simulink model "dynamics_standard_block_CHECK"  (R2017b)
settings: Solver=ode45  StartTime=0.0  StopTime=10  RelTol=1e-3  EnableMultiTasking=on
settings Model: Creator=sagl_ma  LastModifiedBy=hazr_sh
settings DataIOCC: LimitDataPoints=on  SaveFormat=Array
settings OptimizationCC: LifeSpan=inf
settings DebuggingCC: SFUnexpectedBacktrackingDiag=warning  SFNoUnconditionalDefaultTransitionDiag=warning  SFExecutionAtInitializationDiag=none
settings HardwareCC: ProdBitPerPointer=32  ProdBitPerSizeT=32  ProdBitPerPtrDiffT=32  ProdLargestAtomicFloat=None  ProdIntDivRoundTo=Undefined  ProdEndianess=Unspecified  ProdWordSize=32  ProdHWDeviceType=32-bit Generic
settings ModelReferenceCC: PropagateSignalLabelsOutOfModel=off
settings CodeAppCC: StateflowObjectComments=on
settings GRTTargetCC: TargetLangStandard=C89/C90 (ANSI)  GeneratePreprocessorConditionals=Disable all
settings ConfigComp: CovMetricSettings=dw  CovHtmlReporting=on  CovSaveCumulativeToWorkspaceVar=on  CovSaveSingleToWorkspaceVar=on  CovExternalEMLEnable=off

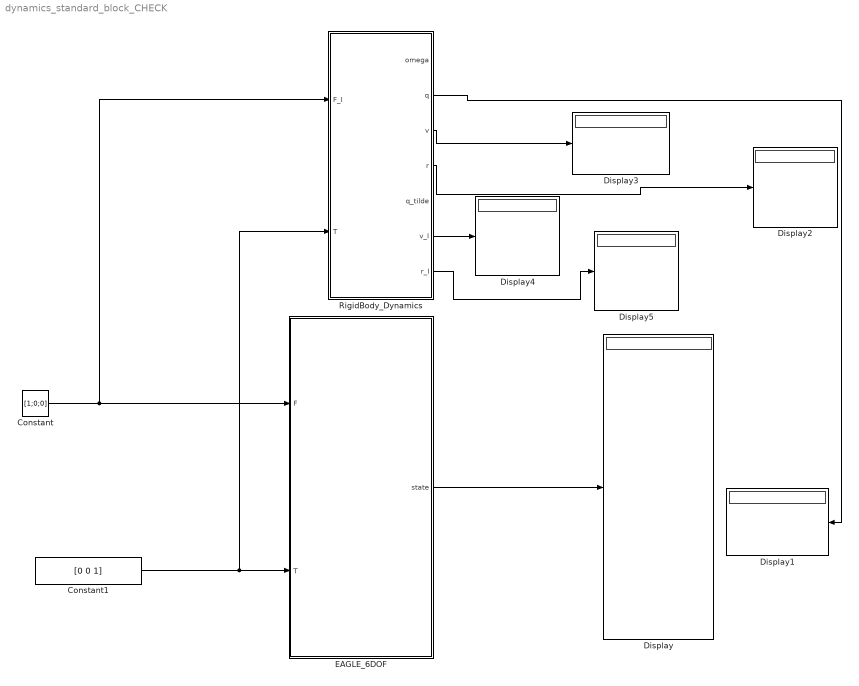
== system dynamics_standard_block_CHECK ==
  Constant : Constant  Value=[1;0;0]
  Constant1 : Constant  Value=[0 0 1]
  Display{,1..5} (6 alike) : Display
  EAGLE_6DOF : Subsystem  mask{r0=[0;0;0], v0=[0;0;0], m0=1, q_I_B0=[0;0;0;1], omega0=[0;0;0], I0=eye(3)}
      mask prompts: r0 "Initial position (m) in inertial reference frame, [3,1]"; v0 "Initial velocity (m/s) in inertial reference frame, [3,1]"; m0 "Initial mass (kg), [1,1]"; q_I_B0 "Initial quaternion defining the orientation from inertial reference frame to body reference frame [4,1]"; omega0 "Initial angular velocity (rad/s) in body reference frame, [3,1]"; I0 "Initial Inertia matrix (kg*m2),  [3,3]"
  RigidBody_Dynamics : Subsystem  mask{r0=[0;0;0], v0=[0;0;0], m0=1, q0=[0;0;0;1], w0=[0;0;0], J0=eye(3)}
      mask prompts: r0 "Initial position (m) in inertial reference frame, [3,1]"; v0 "Initial velocity (m/s) in inertial reference frame, [3,1]"; m0 "Initial mass (kg), [1,1]"; q0 "Initial quaternion defining the orientation in body reference frame [4,1]"; w0 "Initial angular velocity (rad/s) in body reference frame, [3,1]"; J0 "Initial Inertia matrix (kg*m2),  [3,3]"
  wires:
  Constant/1 -> RigidBody_Dynamics/1(F_I), EAGLE_6DOF/1(F)
  Constant1/1 -> RigidBody_Dynamics/2(T), EAGLE_6DOF/2(T)
  EAGLE_6DOF/1(state) -> Display/1
  RigidBody_Dynamics/2(q) -> Display1/1
  RigidBody_Dynamics/4(r) -> Display2/1
  RigidBody_Dynamics/3(v) -> Display3/1
  RigidBody_Dynamics/6("v_I ") -> Display4/1
  RigidBody_Dynamics/7(r_I) -> Display5/1

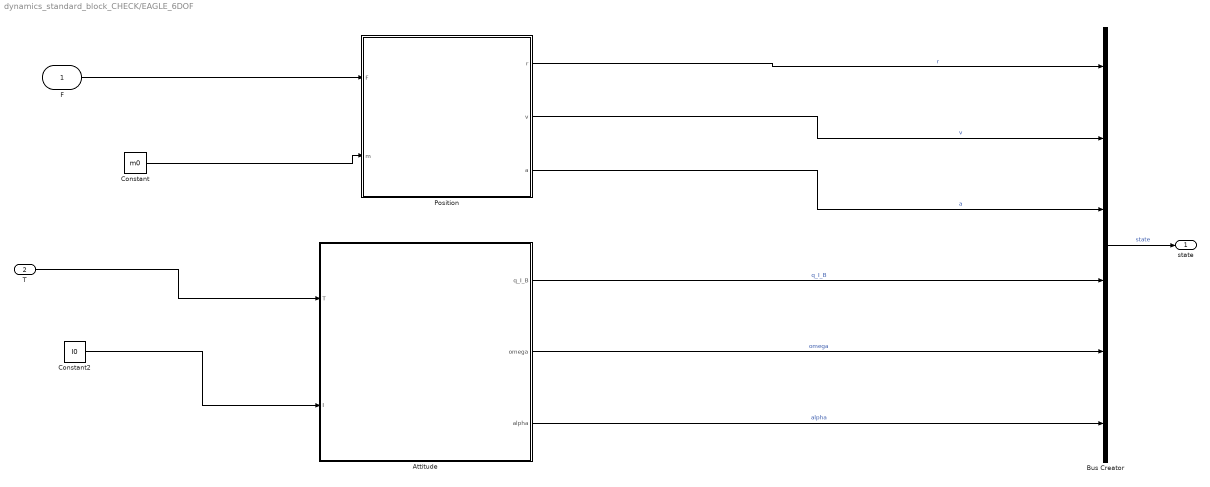
== system dynamics_standard_block_CHECK/EAGLE_6DOF ==
  F : Inport
  T : Inport  Port=2
  Attitude : Subsystem
  Bus Creator : BusCreator  Inputs=6
  Constant : Constant  Value=m0
  Constant2 : Constant  Value=I0
  Position : Subsystem
  state : Outport
  wires:
  Constant2/1 -> Attitude/2(I)
  Attitude/3(alpha) -> Bus Creator/6  "alpha"
  Attitude/2(omega) -> Bus Creator/5  "omega"
  Attitude/1(q_I_B) -> Bus Creator/4  "q_I_B"
  Position/3(a) -> Bus Creator/3  "a"
  Position/1(r) -> Bus Creator/1  "r"
  Position/2(v) -> Bus Creator/2  "v"
  Bus Creator/1 -> state/1  "state"
  Constant/1 -> Position/2(m)
  F/1 -> Position/1(F)
  T/1 -> Attitude/1(T)

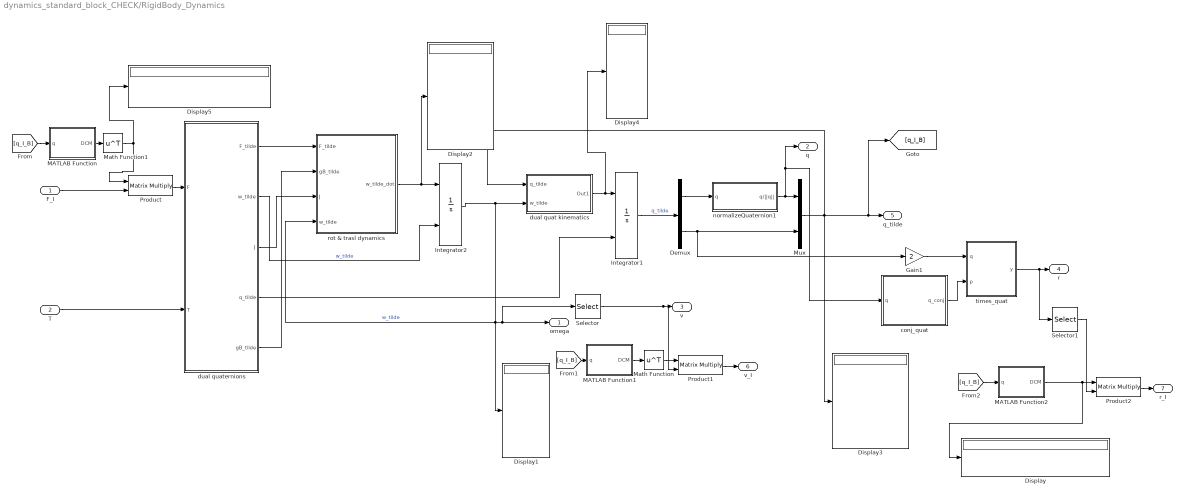
== system dynamics_standard_block_CHECK/RigidBody_Dynamics ==
  F_I : Inport
  T : Inport  Port=2
  Demux : Demux  Outputs=2
  Display{,1..5} (6 alike) : Display
  Gain1 : Gain  Gain=2
  Integrator1 : Integrator  InitialConditionSource=external
  Integrator2 : Integrator  InitialConditionSource=external
  MATLAB Function : MATLAB Function  TreatAsAtomicUnit=on
  MATLAB Function1 : MATLAB Function  TreatAsAtomicUnit=on
  MATLAB Function2 : MATLAB Function  TreatAsAtomicUnit=on
  Math Function : Math  Operator=transpose  SaturateOnIntegerOverflow=on
  Math Function1 : Math  Operator=transpose  SaturateOnIntegerOverflow=on
  Mux : Mux  Inputs=[4,4]
  Product : Product  Multiplication=Matrix(*)
  Product1 : Product  Multiplication=Matrix(*)
  Product2 : Product  Multiplication=Matrix(*)
  Selector : Selector  InputPortWidth=8  IndexOptions=Index vector (dialog)  Indices=[5:7]  OutputSizes=1
  Selector1 : Selector  InputPortWidth=4  IndexOptions=Index vector (dialog)  Indices=[1:3]  OutputSizes=1
  conj_quat : MATLAB Function  TreatAsAtomicUnit=on
  dual quat kinematics : Subsystem
  dual quaternions : Subsystem
  normalizeQuaternion1 : Subsystem  mask(normalizeQuaternion){}
      mask help:
      | This block is normalizing a quaternion. It changes a any quaternion into a
      | unit quaternion.
      |
      | Input:
      | 1) four dimensional quaternion
      |
      | Output:
      | 1) four dimensional unit quaternion
      mask Help: web(which('HPS_mathematics_lib-normalizeQuaternion.html'),'-helpbrowser')
  rot & trasl dynamics : Subsystem
  times_quat : MATLAB Function  TreatAsAtomicUnit=on
  omega : Outport
  q : Outport  Port=2
  v : Outport  Port=3
  r : Outport  Port=4
  "q_tilde " : Outport  Port=5
  "v_I " : Outport  Port=6
  r_I : Outport  Port=7
  wires:
  dual quaternions/1(F_tilde) -> rot & trasl dynamics/1(F_tilde)
  dual quaternions/5(gB_tilde) -> rot & trasl dynamics/2(gB_tilde)
  dual quaternions/3(J) -> rot & trasl dynamics/3(J)
  rot & trasl dynamics/1(w_tilde_dot) -> Display2/1, Integrator2/1
  Integrator2/1 -> Display1/1, Selector/1, omega/1, rot & trasl dynamics/4(w_tilde), dual quat kinematics/2(w_tilde)  "w_tilde"
  dual quat kinematics/1(Out1) -> Display4/1, Integrator1/1
  dual quaternions/2(w_tilde) -> Integrator2/2  "w_tilde"
  dual quaternions/4(q_tilde) -> Integrator1/2
  Demux/1 -> normalizeQuaternion1/1(q)
  Integrator1/1 -> Demux/1  "q_tilde"
  Demux/2 -> Gain1/1, Mux/2
  Gain1/1 -> times_quat/1(q)
  Mux/1 -> dual quat kinematics/1(q_tilde), Display3/1, "q_tilde "/1, [q_I_B]
  [q_I_B] -> MATLAB Function/1(q)
  F_I/1 -> Product/2
  Product/1 -> dual quaternions/1(F)
  normalizeQuaternion1/1(q/||q||) -> conj_quat/1(q), q/1, Mux/1
  conj_quat/1(q_conj) -> times_quat/2(p)
  times_quat/1(y) -> Selector1/1, r/1
  [q_I_B] -> MATLAB Function1/1(q)
  MATLAB Function1/1(DCM) -> Math Function/1
  Selector/1 -> Product1/2, v/1
  Math Function/1 -> Product1/1
  Product1/1 -> "v_I "/1
  [q_I_B] -> MATLAB Function2/1(q)
  Product2/1 -> r_I/1
  Selector1/1 -> Product2/2
  MATLAB Function2/1(DCM) -> Display/1, Product2/1
  MATLAB Function/1(DCM) -> Math Function1/1
  Math Function1/1 -> Product/1, Display5/1
  T/1 -> dual quaternions/2(T)

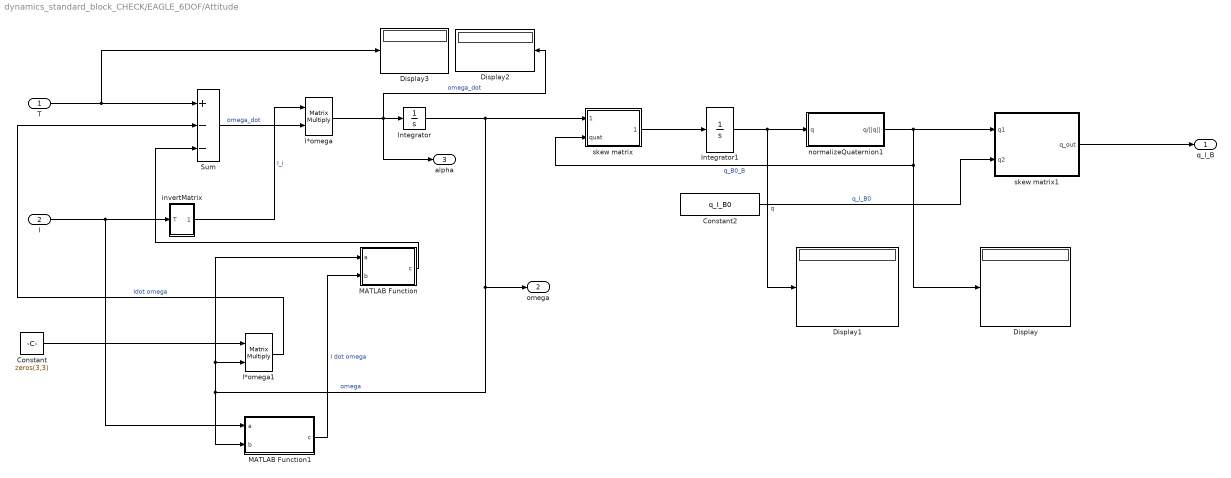
== system dynamics_standard_block_CHECK/EAGLE_6DOF/Attitude ==
  T : Inport
  I : Inport  Port=2
  Constant : Constant  Value=zeros(3,3)
  Constant2 : Constant  Value=q_I_B0
  Display{,1..3} (4 alike) : Display
  I*omega : Product  Multiplication=Matrix(*)  RndMeth=Zero
  I*omega1 : Product  Multiplication=Matrix(*)  RndMeth=Zero
  Integrator : Integrator  InitialCondition=omega0
  Integrator1 : Integrator  InitialCondition=[0;0;0;1]
  MATLAB Function : MATLAB Function  TreatAsAtomicUnit=on
  MATLAB Function1 : MATLAB Function  TreatAsAtomicUnit=on
  Sum : Sum  Inputs=+--
  invertMatrix : Subsystem  mask(invertMatrix){}
      mask help:
      | This block inverts a matrix.
      |
      | Input:
      |     T: [3 x 3] matrix
      |
      | Output:
      |     T_inv: [3 x 3] inverted matrix
      mask Help: web(which('HPS_mathematics_lib-invertMatrix.html'),'-helpbrowser')
  normalizeQuaternion1 : Subsystem  mask(normalizeQuaternion){}
      mask help:
      | This block is normalizing a quaternion. It changes a any quaternion into a
      | unit quaternion.
      |
      | Input:
      | 1) four dimensional quaternion
      |
      | Output:
      | 1) four dimensional unit quaternion
      mask Help: web(which('HPS_mathematics_lib-normalizeQuaternion.html'),'-helpbrowser')
  skew matrix : MATLAB Function  TreatAsAtomicUnit=on
  skew matrix1 : MATLAB Function  TreatAsAtomicUnit=on
  q_I_B : Outport
  omega : Outport  Port=2
  alpha : Outport  Port=3
  wires:
  skew matrix1/1(q_out) -> q_I_B/1
  Constant2/1 -> skew matrix1/2(q2)  "q_I_B0"
  skew matrix/1(quat_dot) -> Integrator1/1
  normalizeQuaternion1/1(q/||q||) -> Display/1, skew matrix/2(quat), skew matrix1/1(q1)  "q_B0_B"
  Integrator1/1 -> Display1/1, normalizeQuaternion1/1(q)  "q"
  Sum/1 -> I*omega/2  "omega_dot"
  MATLAB Function/1(c) -> Sum/3
  MATLAB Function1/1(c) -> MATLAB Function/2(b)  "I dot omega"
  I*omega1/1 -> Sum/2  "Idot omega"
  Constant/1 -> I*omega1/1
  I*omega/1 -> Display2/1, Integrator/1, alpha/1  "omega_dot"
  invertMatrix/1(T_inv) -> I*omega/1  "I_i"
  I/1 -> invertMatrix/1(T), MATLAB Function1/1(a)
  Integrator/1 -> skew matrix/1(omega), omega/1, MATLAB Function1/2(b), I*omega1/2, MATLAB Function/1(a)  "omega"
  T/1 -> Display3/1, Sum/1

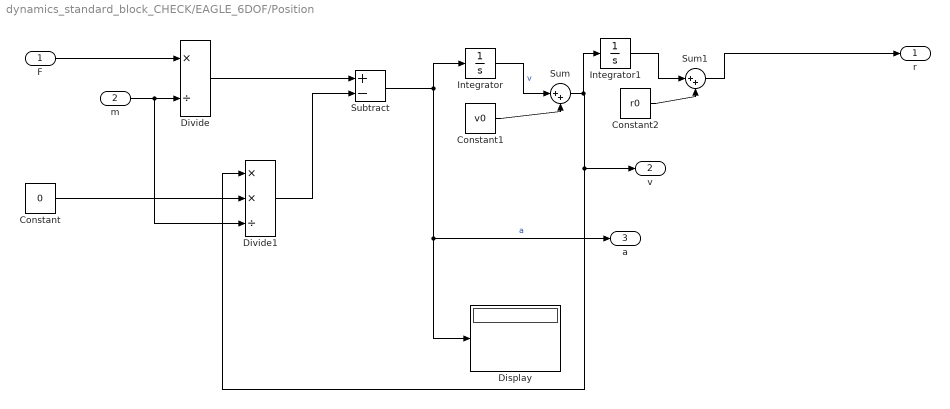
== system dynamics_standard_block_CHECK/EAGLE_6DOF/Position ==
  F : Inport
  m : Inport  Port=2
  Constant : Constant  Value=0
  Constant1 : Constant  Value=v0
  Constant2 : Constant  Value=r0
  Display : Display
  Divide : Product  Inputs=*/
  Divide1 : Product  Inputs=**/
  Integrator : Integrator
  Integrator1 : Integrator
  Subtract : Sum  Inputs=+-
  Sum : Sum  Inputs=|++
  Sum1 : Sum  Inputs=|++
  r : Outport
  v : Outport  Port=2
  a : Outport  Port=3
  wires:
  Sum1/1 -> r/1
  Constant2/1 -> Sum1/2
  Sum/1 -> Divide1/1, v/1, Integrator1/1
  Constant1/1 -> Sum/2
  Subtract/1 -> Display/1, a/1, Integrator/1  "a"
  Integrator/1 -> Sum/1  "v"
  Integrator1/1 -> Sum1/1
  Divide1/1 -> Subtract/2
  Divide/1 -> Subtract/1
  F/1 -> Divide/1
  m/1 -> Divide/2, Divide1/3
  Constant/1 -> Divide1/2

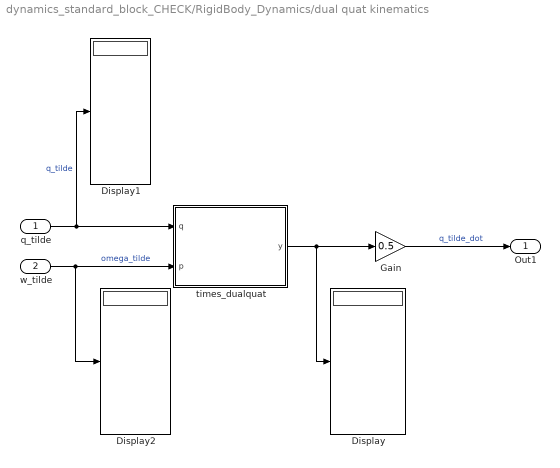
== system dynamics_standard_block_CHECK/RigidBody_Dynamics/dual quat kinematics ==
  q_tilde : Inport
  w_tilde : Inport  Port=2
  Display : Display
  Display1 : Display
  Display2 : Display
  Gain : Gain  Gain=0.5
  times_dualquat : MATLAB Function  TreatAsAtomicUnit=on
  Out1 : Outport
  wires:
  q_tilde/1 -> Display1/1, times_dualquat/1(q)  "q_tilde"
  w_tilde/1 -> Display2/1, times_dualquat/2(p)  "omega_tilde"
  times_dualquat/1(y) -> Display/1, Gain/1
  Gain/1 -> Out1/1  "q_tilde_dot"

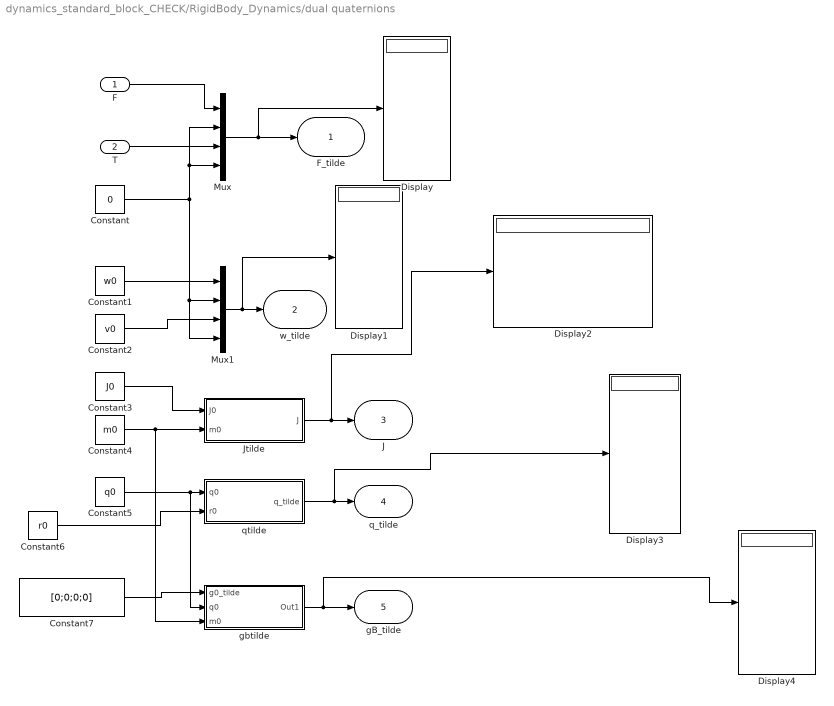
== system dynamics_standard_block_CHECK/RigidBody_Dynamics/dual quaternions ==
  F : Inport
  T : Inport  Port=2
  Constant : Constant  Value=0
  Constant1 : Constant  Value=w0  VectorParams1D=off
  Constant2 : Constant  Value=v0  VectorParams1D=off
  Constant3 : Constant  Value=J0
  Constant4 : Constant  Value=m0  VectorParams1D=off
  Constant5 : Constant  Value=q0  VectorParams1D=off
  Constant6 : Constant  Value=r0  VectorParams1D=off
  Constant7 : Constant  Value=[0;0;0;0]  VectorParams1D=off
  Display{,1..4} (5 alike) : Display
  Jtilde : Subsystem
  Mux : Mux
  Mux1 : Mux
  gbtilde : Subsystem
  qtilde : Subsystem
  F_tilde : Outport
  w_tilde : Outport  Port=2
  J : Outport  Port=3
  q_tilde : Outport  Port=4
  gB_tilde : Outport  Port=5
  wires:
  F/1 -> Mux/1
  Constant/1 -> Mux1/2, Mux1/4, Mux/2, Mux/4
  Constant3/1 -> Jtilde/1(J0)
  Constant1/1 -> Mux1/1
  Constant5/1 -> gbtilde/2("q0 "), qtilde/1(q0)
  Mux/1 -> Display/1, F_tilde/1
  Mux1/1 -> Display1/1, w_tilde/1
  Constant2/1 -> Mux1/3
  Constant7/1 -> gbtilde/1(g0_tilde)
  Constant6/1 -> qtilde/2(r0)
  Constant4/1 -> Jtilde/2("m0 "), gbtilde/3(m0)
  T/1 -> Mux/3
  Jtilde/1(J) -> Display2/1, J/1
  qtilde/1(q_tilde) -> Display3/1, q_tilde/1
  gbtilde/1(Out1) -> Display4/1, gB_tilde/1

== system dynamics_standard_block_CHECK/RigidBody_Dynamics/normalizeQuaternion1 ==
  q : Inport
  HPS_normalizeQuaternion : MATLAB Function  TreatAsAtomicUnit=on
  q/||q|| : Outport
  wires:
  q/1 -> HPS_normalizeQuaternion/1(q)
  HPS_normalizeQuaternion/1(qOut) -> q/||q||/1

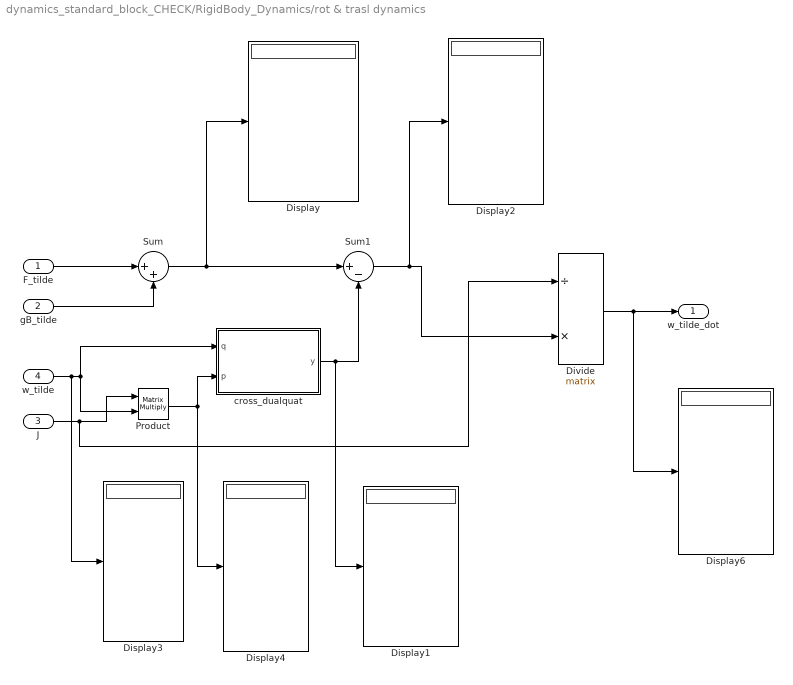
== system dynamics_standard_block_CHECK/RigidBody_Dynamics/rot & trasl dynamics ==
  F_tilde : Inport
  gB_tilde : Inport  Port=2
  J : Inport  Port=3
  w_tilde : Inport  Port=4
  Display{,1..4,6} (6 alike) : Display
  Divide : Product  Inputs=/*  Multiplication=Matrix(*)
  Product : Product  Multiplication=Matrix(*)
  Sum : Sum  Inputs=|++
  Sum1 : Sum  Inputs=|+-
  cross_dualquat : MATLAB Function  TreatAsAtomicUnit=on
  w_tilde_dot : Outport
  wires:
  F_tilde/1 -> Sum/1
  gB_tilde/1 -> Sum/2
  J/1 -> Divide/1, Product/1
  w_tilde/1 -> Display3/1, cross_dualquat/1(q), Product/2
  Sum/1 -> Sum1/1, Display/1
  cross_dualquat/1(y) -> Sum1/2, Display1/1
  Product/1 -> cross_dualquat/2(p), Display4/1
  Sum1/1 -> Display2/1, Divide/2
  Divide/1 -> Display6/1, w_tilde_dot/1

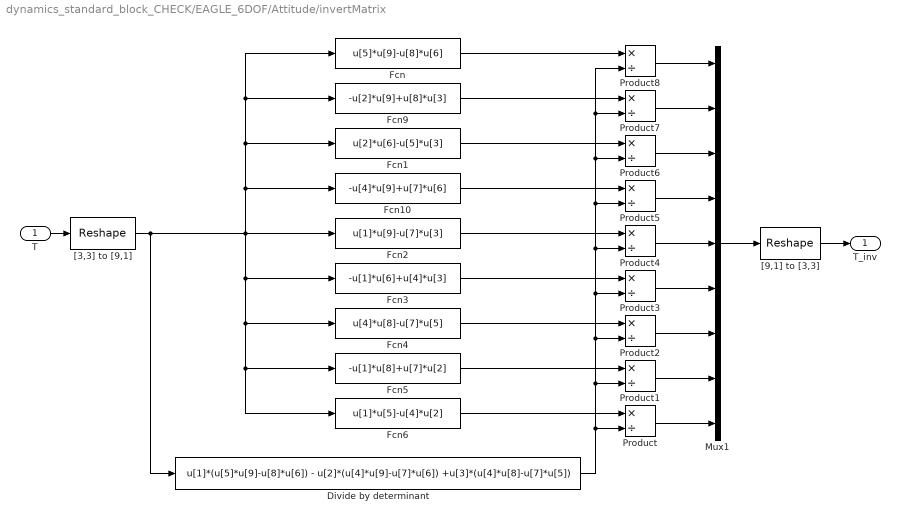
== system dynamics_standard_block_CHECK/EAGLE_6DOF/Attitude/invertMatrix ==
  T : Inport
  Divide by determinant : Fcn  Expr=u[1]*(u[5]*u[9]-u[8]*u[6]) - u[2]*(u[4]*u[9]-u[7]*u[6]) +u[3]*(u[4]*u[8]-u[7]*u[5])
  Fcn : Fcn  Expr=u[5]*u[9]-u[8]*u[6]
  Fcn1 : Fcn  Expr=u[2]*u[6]-u[5]*u[3]
  Fcn10 : Fcn  Expr=-u[4]*u[9]+u[7]*u[6]
  Fcn2 : Fcn  Expr=u[1]*u[9]-u[7]*u[3]
  Fcn3 : Fcn  Expr=-u[1]*u[6]+u[4]*u[3]
  Fcn4 : Fcn  Expr=u[4]*u[8]-u[7]*u[5]
  Fcn5 : Fcn  Expr=-u[1]*u[8]+u[7]*u[2]
  Fcn6 : Fcn  Expr=u[1]*u[5]-u[4]*u[2]
  Fcn9 : Fcn  Expr=-u[2]*u[9]+u[8]*u[3]
  Mux1 : Mux  Inputs=9
  Product{,1..8} (9 alike) : Product  Inputs=*/  SaturateOnIntegerOverflow=on  InputSameDT=on  OutDataTypeStr=Inherit: Same as first input
  "[3,3] to [9,1]" : Reshape  OutputDimensionality=Customize  OutputDimensions=[9,1]
  "[9,1] to [3,3]" : Reshape  OutputDimensionality=Customize  OutputDimensions=[3,3]
  T_inv : Outport
  wires:
  Mux1/1 -> "[9,1] to [3,3]"/1
  "[3,3] to [9,1]"/1 -> Divide by determinant/1, Fcn/1, Fcn9/1, Fcn1/1, Fcn10/1, Fcn2/1, Fcn3/1, Fcn4/1, Fcn5/1, Fcn6/1
  Divide by determinant/1 -> Product/2, Product8/2, Product7/2, Product6/2, Product5/2, Product4/2, Product3/2, Product2/2, Product1/2
  Product7/1 -> Mux1/2
  Product6/1 -> Mux1/3
  Product5/1 -> Mux1/4
  Product4/1 -> Mux1/5
  Fcn/1 -> Product8/1
  Product/1 -> Mux1/9
  "[9,1] to [3,3]"/1 -> T_inv/1
  T/1 -> "[3,3] to [9,1]"/1
  Fcn9/1 -> Product7/1
  Fcn1/1 -> Product6/1
  Fcn10/1 -> Product5/1
  Fcn2/1 -> Product4/1
  Product1/1 -> Mux1/8
  Product2/1 -> Mux1/7
  Product3/1 -> Mux1/6
  Fcn3/1 -> Product3/1
  Fcn4/1 -> Product2/1
  Fcn5/1 -> Product1/1
  Fcn6/1 -> Product/1
  Product8/1 -> Mux1/1

== system dynamics_standard_block_CHECK/EAGLE_6DOF/Attitude/normalizeQuaternion1 ==
  q : Inport
  HPS_normalizeQuaternion : MATLAB Function  TreatAsAtomicUnit=on
  q/||q|| : Outport
  wires:
  q/1 -> HPS_normalizeQuaternion/1(q)
  HPS_normalizeQuaternion/1(qOut) -> q/||q||/1

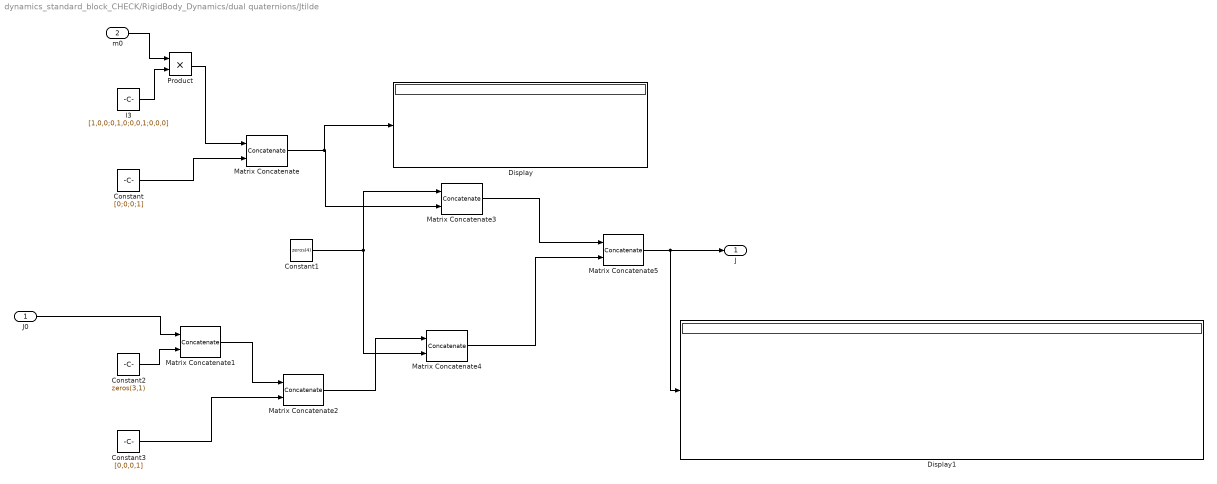
== system dynamics_standard_block_CHECK/RigidBody_Dynamics/dual quaternions/Jtilde ==
  J0 : Inport
  "m0 " : Inport  Port=2
  Constant : Constant  Value=[0;0;0;1]  VectorParams1D=off
  Constant1 : Constant  Value=zeros(4)
  Constant2 : Constant  Value=zeros(3,1)
  Constant3 : Constant  Value=[0,0,0,1]  VectorParams1D=off
  Display : Display
  Display1 : Display
  I3 : Constant  Value=[1,0,0;0,1,0;0,0,1;0,0,0]
  Matrix Concatenate{,1,3..4} (4 alike) : Concatenate  Mode=Multidimensional array  ConcatenateDimension=2
  Matrix Concatenate2 : Concatenate  Mode=Multidimensional array
  Matrix Concatenate5 : Concatenate  Mode=Multidimensional array
  Product : Product
  J : Outport
  wires:
  Constant/1 -> Matrix Concatenate/2
  J0/1 -> Matrix Concatenate1/1
  Constant2/1 -> Matrix Concatenate1/2
  Matrix Concatenate1/1 -> Matrix Concatenate2/1
  Constant1/1 -> Matrix Concatenate4/2, Matrix Concatenate3/1
  Matrix Concatenate/1 -> Display/1, Matrix Concatenate3/2
  Matrix Concatenate2/1 -> Matrix Concatenate4/1
  Matrix Concatenate3/1 -> Matrix Concatenate5/1
  Matrix Concatenate4/1 -> Matrix Concatenate5/2
  I3/1 -> Product/2
  Product/1 -> Matrix Concatenate/1
  Constant3/1 -> Matrix Concatenate2/2
  Matrix Concatenate5/1 -> Display1/1, J/1
  "m0 "/1 -> Product/1

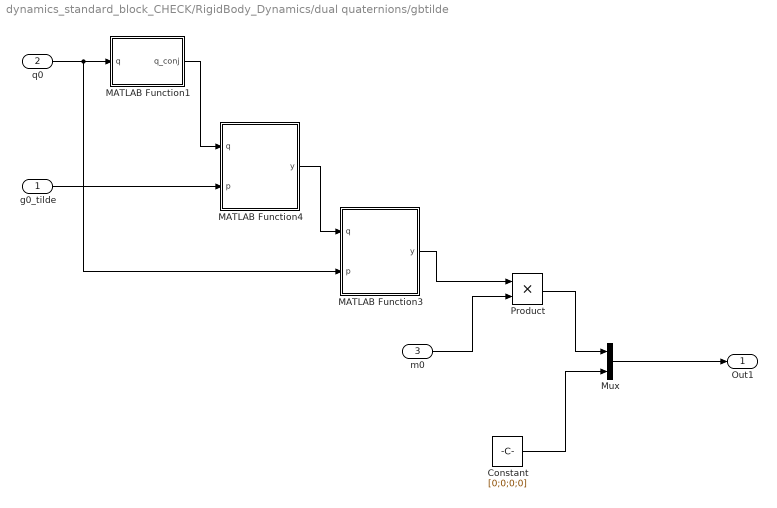
== system dynamics_standard_block_CHECK/RigidBody_Dynamics/dual quaternions/gbtilde ==
  g0_tilde : Inport
  "q0 " : Inport  Port=2
  m0 : Inport  Port=3
  Constant : Constant  Value=[0;0;0;0]  VectorParams1D=off
  MATLAB Function1 : MATLAB Function  TreatAsAtomicUnit=on
  MATLAB Function3 : MATLAB Function  TreatAsAtomicUnit=on
  MATLAB Function4 : MATLAB Function  TreatAsAtomicUnit=on
  Mux : Mux  Inputs=2
  Product : Product
  Out1 : Outport
  wires:
  "q0 "/1 -> MATLAB Function3/2(p), MATLAB Function1/1(q)
  g0_tilde/1 -> MATLAB Function4/2(p)
  MATLAB Function3/1(y) -> Product/1
  Product/1 -> Mux/1
  Constant/1 -> Mux/2
  Mux/1 -> Out1/1
  MATLAB Function1/1(q_conj) -> MATLAB Function4/1(q)
  m0/1 -> Product/2
  MATLAB Function4/1(y) -> MATLAB Function3/1(q)

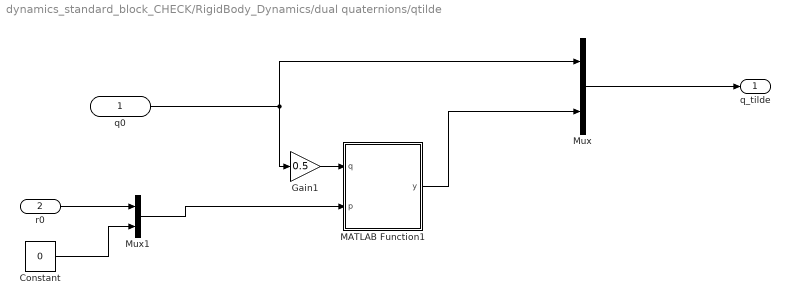
== system dynamics_standard_block_CHECK/RigidBody_Dynamics/dual quaternions/qtilde ==
  q0 : Inport
  r0 : Inport  Port=2
  Constant : Constant  Value=0
  Gain1 : Gain  Gain=0.5
  MATLAB Function1 : MATLAB Function  TreatAsAtomicUnit=on
  Mux : Mux  Inputs=2
  Mux1 : Mux  Inputs=2
  q_tilde : Outport
  wires:
  q0/1 -> Gain1/1, Mux/1
  Mux/1 -> q_tilde/1
  Constant/1 -> Mux1/2
  r0/1 -> Mux1/1
  MATLAB Function1/1(y) -> Mux/2
  Mux1/1 -> MATLAB Function1/2(p)
  Gain1/1 -> MATLAB Function1/1(q)

== matlab function dynamics_standard_block_CHECK/RigidBody_Dynamics/dual quaternions/gbtilde/MATLAB Function1 ==
  data: q input; q_conj output
function q_conj = conj_quat(q)
%Unit quaternion conjugation

q0= q(4);
q_vect= q(1:3);

q_conj = [-q_vect; q0];

== matlab function dynamics_standard_block_CHECK/RigidBody_Dynamics/dual quat kinematics/times_dualquat ==
  data: q input; y output; p input
function y = times_dualquat(q,p)
% Dual Quaternion Cross Product

q1= q(1:4);
q10= q1(4);
q1vect= q1(1:3);

p1= p(1:4);
p10= p1(4);
p1vect= p1(1:3);

q2= q(5:8);
q20= q2(4);
q2vect= q2(1:3);

p2= p(5:8);
p20= p2(4);
p2vect= p2(1:3);

y1= [q10.*p1vect + p10.*q1vect + cross(q1vect, p1vect); ...
    q10*p10 - q1vect'*p1vect];
y2= [q10.*p2vect + p20.*q1vect + cross(q1vect, p2vect); ...
    q10*p20 - q1vect'*p2vect];
y3= [q20.*p1vect + p10.*q2vect + cross(q2vect, p1vect); ...
    q20*p10 - q2vect'*p1vect];

y= [y1; y2+y3];

== matlab function dynamics_standard_block_CHECK/EAGLE_6DOF/Attitude/MATLAB Function ==
  data: a input; c output; b input
function c = cross_prod(a,b)
%#codegen

% c = a cross b

c = cross(a,b);

== matlab function dynamics_standard_block_CHECK/EAGLE_6DOF/Attitude/MATLAB Function1 ==
  data: a input; c output; b input
function c = matrix_dot_prod(a,b)
%#codegen

% c = a * b

c = a*b;

== matlab function dynamics_standard_block_CHECK/RigidBody_Dynamics/dual quaternions/gbtilde/MATLAB Function4 ==
  data: q input; y output; p input
function y = times_quat(q,p)
% Quaternion multiplication 

q0= q(4);
p0= p(4);

q_vect= q(1:3);
p_vect= p(1:3);


y = [q0.*p_vect + p0.*q_vect + cross(q_vect, p_vect); ...
    q0*p0 - sum(q_vect.*p_vect,1)];

== matlab function dynamics_standard_block_CHECK/RigidBody_Dynamics/dual quaternions/qtilde/MATLAB Function1 ==
  data: q input; y output; p input
function y = times_quat(q,p)
% Quaternion multiplication 

q0= q(4);
p0= p(4);

q_vect= q(1:3);
p_vect= p(1:3);


y = [q0.*p_vect + p0.*q_vect + cross(q_vect, p_vect); ...
    q0*p0 - sum(q_vect.*p_vect,1)];

== matlab function dynamics_standard_block_CHECK/RigidBody_Dynamics/normalizeQuaternion1/HPS_normalizeQuaternion ==
  data: q input; qOut output
%----------------------------------------------------------------------------
%
%            High Performance Satellite Dynamics Simulator (HPS)
%        (c) copyright 2001 - 2008 ZARM, University of Bremen
%        (c) copyright 2008 - 2012 ZARM, University of Bremen
%        and Institute of Space Systems, DLR e.V.
%
%----------------------------------------------------------------------------
%% normalizeQuaternion()
%
% * $LastChangedBy$
% * $LastChangedRevision$
% * $LastChangedDate$
%
% *Change Record:*
%
% * 2009/10/13      - Ansgar Heidecker, initial realease
% * 2010/07/02      - Ansgar Heidecker, moved file from AF/SSB to HPS
% * 2014/10/24      - Stephen Steffes, allowed for array inputs
%
%%%
% This block normalizes a quaternion using the vector norm.
% Its basis is the embedded Matlab function
% \textit{HPS\_normalizeQuaternion.m} that is wrapped into the Simulink
% block.  If the input is a zero quaternion, the output is also a zero
% quaternion.
% 
% The inputs can be single quaternions in row or column form, or arrays
% of quaternions in column form. I.e. the size of $q$ is either $4xN$ or
% $1x4$.
% 
% *Inputs:*
% 
% * q - [4xN or 1x4] Vector or array of quaternion columns
% 
% *Returns:*
% 
% * qOut - [4xN or 1x4] Normalized quaternions with the same size as the input.
%

function qOut = HPS_normalizeQuaternion(q)
%#codegen
%#eml

    sz=size(q); %sz(1)= #rows, sz(2)= #columns
    if( (sz(1)==1 && sz(2)==4) ) % q is row vector
        n=norm(q);
        if(n~=0) % protect from div-by-0
            qOut=q/norm(q);
        else
            qOut=q;
        end
    elseif( sz(1)~=4 ) % size of q is invalid
        error('ErrorTests:convertTest','Invalid size of q.\nEither #rows of q ~= 4 or q is not a row vector with 4 cols.');
    else
        n=sqrt(sum(q.^2));
        n=n+(n==0); % protect from div-by-0
        qOut=q./(ones(4,1)*n);
    end
end

%% Reference
%
% * Wertz J.R., Spacecraft Attitude Determination and Control, Reprint
% 2002, Kluwer Academic Publishers, Appendix D

== matlab function dynamics_standard_block_CHECK/RigidBody_Dynamics/dual quaternions/gbtilde/MATLAB Function3 ==
  data: q input; y output; p input
function y = times_quat(q,p)
% Quaternion multiplication 

q0= q(4);
p0= p(4);

q_vect= q(1:3);
p_vect= p(1:3);


y = [q0.*p_vect + p0.*q_vect + cross(q_vect, p_vect); ...
    q0*p0 - sum(q_vect.*p_vect,1)];

== matlab function dynamics_standard_block_CHECK/EAGLE_6DOF/Attitude/normalizeQuaternion1/HPS_normalizeQuaternion ==
  data: q input; qOut output
%----------------------------------------------------------------------------
%
%            High Performance Satellite Dynamics Simulator (HPS)
%        (c) copyright 2001 - 2008 ZARM, University of Bremen
%        (c) copyright 2008 - 2012 ZARM, University of Bremen
%        and Institute of Space Systems, DLR e.V.
%
%----------------------------------------------------------------------------
%% normalizeQuaternion()
%
% * $LastChangedBy$
% * $LastChangedRevision$
% * $LastChangedDate$
%
% *Change Record:*
%
% * 2009/10/13      - Ansgar Heidecker, initial realease
% * 2010/07/02      - Ansgar Heidecker, moved file from AF/SSB to HPS
% * 2014/10/24      - Stephen Steffes, allowed for array inputs
%
%%%
% This block normalizes a quaternion using the vector norm.
% Its basis is the embedded Matlab function
% \textit{HPS\_normalizeQuaternion.m} that is wrapped into the Simulink
% block.  If the input is a zero quaternion, the output is also a zero
% quaternion.
% 
% The inputs can be single quaternions in row or column form, or arrays
% of quaternions in column form. I.e. the size of $q$ is either $4xN$ or
% $1x4$.
% 
% *Inputs:*
% 
% * q - [4xN or 1x4] Vector or array of quaternion columns
% 
% *Returns:*
% 
% * qOut - [4xN or 1x4] Normalized quaternions with the same size as the input.
%

function qOut = HPS_normalizeQuaternion(q)
%#codegen
%#eml

    sz=size(q);
    if( (sz(1)==1 && sz(2)==4) ) % q is row vector
        n=norm(q);
        if(n~=0) % protect from div-by-0
            qOut=q/norm(q);
        else
            qOut=q;
        end
    elseif( sz(1)~=4 ) % size of q is invalid
        error('ErrorTests:convertTest','Invalid size of q.\nEither #rows of q ~= 4 or q is not a row vector with 4 cols.');
    else
        n=sqrt(sum(q.^2));
        n=n+(n==0); % protect from div-by-0
        qOut=q./(ones(4,1)*n);
    end
end

%% Reference
%
% * Wertz J.R., Spacecraft Attitude Determination and Control, Reprint
% 2002, Kluwer Academic Publishers, Appendix D

== matlab function dynamics_standard_block_CHECK/RigidBody_Dynamics/rot & trasl dynamics/cross_dualquat ==
  data: q input; y output; p input
function y = cross_dualquat(q,p)
% Dual Quaternion Cross Product

q1= q(1:4);
q10= q1(4);
q1vect= q1(1:3);

p1= p(1:4);
p10= p1(4);
p1vect= p1(1:3);

q2= q(5:8);
q20= q2(4);
q2vect= q2(1:3);

p2= p(5:8);
p20= p2(4);
p2vect= p2(1:3);

y1= [q10.*p1vect + p10.*q1vect + cross(q1vect, p1vect); 0];
y2= [q10.*p2vect + p20.*q1vect + cross(q1vect, p2vect); 0];
y3= [q20.*p1vect + p10.*q2vect + cross(q2vect, p1vect); 0];

y= [y1; y2+y3];

== matlab function dynamics_standard_block_CHECK/EAGLE_6DOF/Attitude/skew matrix ==
  data: omega input; quat_dot output; quat input
function quat_dot = fcn(omega,quat)
%#codegen

p = omega(1);
q = omega(2);
r = omega(3);
OMEGA = zeros(4,4);
OMEGA = .5*[0 r -q p; -r 0 p q; q -p 0 r; -p -q -r 0];

quat_dot = OMEGA*quat;

return

== matlab function dynamics_standard_block_CHECK/EAGLE_6DOF/Attitude/skew matrix1 ==
  data: q1 input; q_out output; q2 input
% q_multiply.m
% Function to multiply two quaternions together using the (x) opperator.  
% The result is the same as multiplying the DCM versions of the quaternions 
% in the same order.  I.E.
% Q2DCM(q_out) = Q2DCM(q1) * Q2DCM(q2) = Q2DCM(q1 (x) q2) = Q2DCM(q_multiply(q1,q2)
%
% Inputs:
%     q1 - Left side quaternions in (vector,scalar) form, array of
%     quaternion columns
%     q2 - Right side quaternion in (vector,scalar) form, array of
%     quaternion columns
%
% Outputs:
%     q_out - Product quaternion in (vector,scalar) form
% 
% Notes:
% See J. R. Wertz, "Spacecraft Attitude Determination and Control", 1978
% eq D-13
function q_out =q_multiply(q1,q2)
%#codegen

sz1=size(q1);
sz2=size(q2);
if((sz1(1) ~= 4)||(sz2(1) ~= 4))
    error('Quaternions must be the columns of the inputs');
end
if(~((sz1(2) == sz2(2)) || (sz1(2) == 1) || (sz2(2) == 1)))
    error('Either #cols of q1==#cols of q2, #cols of q1==1 or #cols of q2==1');
end

q_out=zeros(4,max([sz1(2) sz2(2)])); %set the size of q_out

q_out(1,:)=q1(4,:).*q2(1,:)+q2(4,:).*q1(1,:)-q1(2,:).*q2(3,:)+q1(3,:).*q2(2,:);
q_out(2,:)=q1(4,:).*q2(2,:)+q2(4,:).*q1(2,:)-q1(3,:).*q2(1,:)+q1(1,:).*q2(3,:);
q_out(3,:)=q1(4,:).*q2(3,:)+q2(4,:).*q1(3,:)-q1(1,:).*q2(2,:)+q1(2,:).*q2(1,:);
q_out(4,:)=q1(4,:).*q2(4,:)-(q1(1,:).*q2(1,:)+q1(2,:).*q2(2,:)+q1(3,:).*q2(3,:));

== matlab function dynamics_standard_block_CHECK/RigidBody_Dynamics/MATLAB Function ==
  data: q input; DCM output
% Q2DCM.m
% Function to convert quaternion to DCM.
%
% Inputs:
%     q - The quaternion to use in (vector,scalar) form
% 
% Outputs:
%     DCM - The DCM representation of q
% 
% Notes:
% See J. R. Wertz, "Spacecraft Attitude Determination and Control", 1978
% eq 12-13
function DCM = Q2DCM(q)
%#eml
q=reshape(q,[],1);

qx=[0 -q(3) q(2);q(3) 0 -q(1);-q(2) q(1) 0];

DCM=(q(4)^2-dot(q(1:3),q(1:3)))*eye(3)+2*q(1:3)*q(1:3)'-2*q(4)*qx;

return

== matlab function dynamics_standard_block_CHECK/RigidBody_Dynamics/conj_quat ==
  data: q input; q_conj output
function q_conj = conj_quat(q)
%Unit quaternion conjugation

q0= q(4);
q_vect= q(1:3);

q_conj = [-q_vect; q0];

== matlab function dynamics_standard_block_CHECK/RigidBody_Dynamics/times_quat ==
  data: q input; y output; p input
function y = times_quat(q,p)
% Quaternion multiplication 

q0= q(4);
p0= p(4);

q_vect= q(1:3);
p_vect= p(1:3);


y = [q0.*p_vect + p0.*q_vect + cross(q_vect, p_vect); ...
    q0*p0 - sum(q_vect.*p_vect,1)];

== matlab function dynamics_standard_block_CHECK/RigidBody_Dynamics/MATLAB Function1 ==
  data: q input; DCM output
% Q2DCM.m
% Function to convert quaternion to DCM.
%
% Inputs:
%     q - The quaternion to use in (vector,scalar) form
% 
% Outputs:
%     DCM - The DCM representation of q
% 
% Notes:
% See J. R. Wertz, "Spacecraft Attitude Determination and Control", 1978
% eq 12-13
function DCM = Q2DCM(q)
%#eml
q=reshape(q,[],1);

qx=[0 -q(3) q(2);q(3) 0 -q(1);-q(2) q(1) 0];

DCM=(q(4)^2-dot(q(1:3),q(1:3)))*eye(3)+2*q(1:3)*q(1:3)'-2*q(4)*qx;

return

== matlab function dynamics_standard_block_CHECK/RigidBody_Dynamics/MATLAB Function2 ==
  data: q input; DCM output
% Q2DCM.m
% Function to convert quaternion to DCM.
%
% Inputs:
%     q - The quaternion to use in (vector,scalar) form
% 
% Outputs:
%     DCM - The DCM representation of q
% 
% Notes:
% See J. R. Wertz, "Spacecraft Attitude Determination and Control", 1978
% eq 12-13
function DCM = Q2DCM(q)
%#eml
q=reshape(q,[],1);

qx=[0 -q(3) q(2);q(3) 0 -q(1);-q(2) q(1) 0];

DCM=(q(4)^2-dot(q(1:3),q(1:3)))*eye(3)+2*q(1:3)*q(1:3)'-2*q(4)*qx;

return
